simulink model "model_hydrau"  (R2022b)
settings: Solver=VariableStepAuto  StartTime=0.0  StopTime=tmax  MaxStep=2  RelTol=1e-3
values from neighbouring files (symbols this model uses):
  dFmw = 0    [obliczenia.m]    (also in obliczenia2.m)
  k1 = (0.329)/0.0050    (= 65.8)    [obliczenia.m]    (also in obliczenia2.m)
  khC = (91.8012 -90)/0.02    (= 90.06)    [obliczenia.m]
  Kp = 0.9*TczasC/(kC*TopuC)    (= 0.165208580467)    [obliczenia.m]    (also in obliczenia2.m = 1.05226274907)
  Tczas1 = 15543 - Topu1 - tsok    (= 12463)    [obliczenia.m]    (also in obliczenia2.m)
  TczashC = 12982 - Topuh - tsok    (= 9758)    [obliczenia.m]
  Ti = 3.33*TopuC/Kp    (= 13061.3070696)    [obliczenia.m]    (also in obliczenia2.m = 11755.1763626)
  Topu1 = 3080 - tsok    (= 1080)    [obliczenia.m]    (also in obliczenia2.m)
  Topuh = 3224 - tsok    (= 1224)    [obliczenia.m]
  TopuhC = 2740 - tsok    (= 740)    [obliczenia.m]
  TozN = TgzN    (= 90)    [obliczenia.m]    (also in obliczenia2.m)
  tsok = 2000    [obliczenia.m]    (also in obliczenia2.m = 80000)
  Twew10 = (Cpw*Fmg10 *Kcg*Tgz10 + Kcw*(Kcg + Cpw*Fmg10)*Tzew0)/(Kcg*Kcw + Cpw*Fmg10*(Kcg + Kcw))    (= 20)    [obliczenia.m]    (also in obliczenia2.m)
undefined symbols (not defined in the file or in its folder): dTwew
libraries: slpidlib x1
settings Model: Creator=asialalala  LastModifiedBy=asialalala
settings DataIOCC: SaveFormat=Array  ReturnWorkspaceOutputs=off

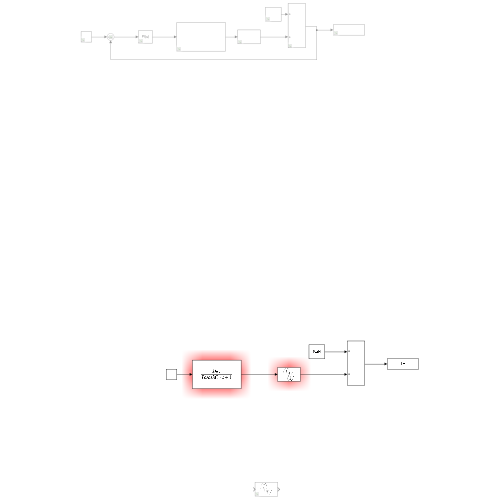
[thumbnail: Simulink's stored preview of the top-level diagram]
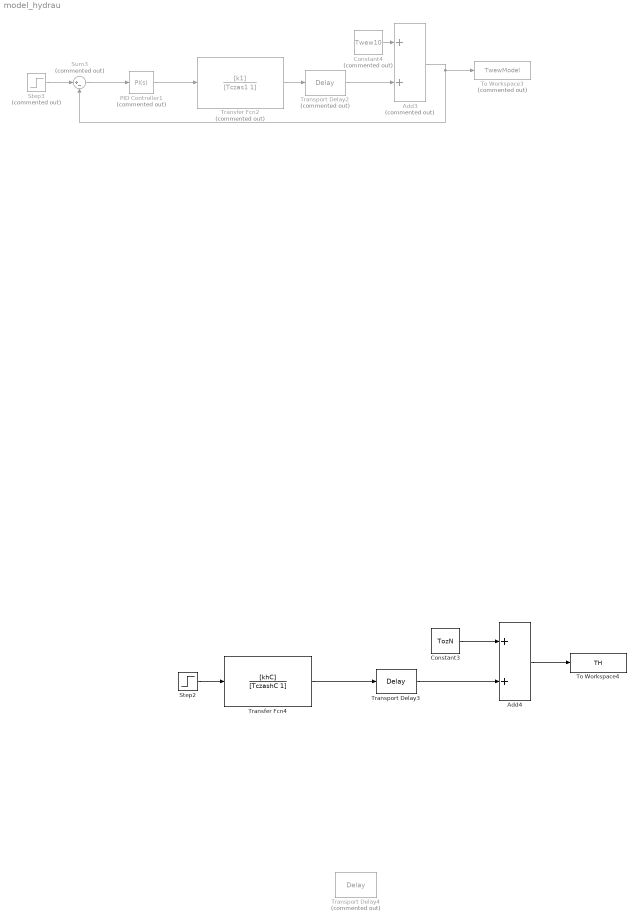
== system model_hydrau ==
  Add3 : Sum  Commented=on
  Add4 : Sum
  Constant3 : Constant  Value=TozN
  Constant4 : Constant  Commented=on  Value=Twew10
  PID Controller1 : slpidlib/PID Controller  Commented=on  Controller=PI  Form=Parallel  TimeDomain=Continuous-time  UseExternalTs=off  SampleTime=-1  IntegratorMethod=Forward Euler  FilterMethod=Forward Euler  ControllerParametersSource=internal  P=Kp  I=1/Ti  UseKiTs=off  D=0  N=100  UseFilter=on  TunerSelectOption=Transfer Function Based (PID Tuner App)  InitialConditionSource=internal  InitialConditionForIntegrator=0  InitialConditionForFilter=0  DifferentiatorICPrevScaledInput=0  ExternalReset=none  TrackingMode=off  Kt=1  LimitOutput=off  SatLimitsSource=internal  UpperSaturationLimit=inf  LowerSaturationLimit=-inf  LinearizeAsGain=on  AntiWindupMode=none  Kb=1  LimitIntegrator=off  UpperIntegratorSaturationLimit=inf  LowerIntegratorSaturationLimit=-inf  POutMin=[]  POutMax=[]  IOutMin=[]  IOutMax=[]  DOutMin=[]  DOutMax=[]  NOutMin=[]  NOutMax=[]  SumOutMin=[]  SumOutMax=[]  SaturationOutMin=[]  SaturationOutMax=[]  PParamMin=[]  PParamMax=[]  IParamMin=[]  IParamMax=[]  DParamMin=[]  DParamMax=[]  NParamMin=[]  NParamMax=[]  KbParamMin=[]  KbParamMax=[]  KtParamMin=[]  KtParamMax=[]  KbOutMin=[]  KbOutMax=[]  KtOutMin=[]  KtOutMax=[]  IntegratorOutMin=[]  IntegratorOutMax=[]  FilterOutMin=[]  FilterOutMax=[]  SumI1OutMin=[]  SumI1OutMax=[]  SumI2OutMin=[]  SumI2OutMax=[]  SumI3OutMin=[]  SumI3OutMax=[]  SumI4OutMin=[]  SumI4OutMax=[]  SumDOutMin=[]  SumDOutMax=[]  DifferentiatorOutMin=[]  DifferentiatorOutMax=[]  FilterDiffOutCoefMin=[]  FilterDiffOutCoefMax=[]  ReciprocalOutMin=[]  ReciprocalOutMax=[]  SumDenOutMin=[]  SumDenOutMax=[]  SumNumOutMin=[]  SumNumOutMax=[]  DivideOutMin=[]  DivideOutMax=[]  UdiffTsProdOutMin=[]  UdiffTsProdOutMax=[]  NTsProdOutMin=[]  NTsProdOutMax=[]  UintegralTsProdOutMin=[]  UintegralTsProdOutMax=[]  UngainTsProdOutMin=[]  UngainTsProdOutMax=[]  ClampingZeroOutDataTypeStr=Inherit: Inherit via back propagation  ClampingZeroOutMin=[]  ClampingZeroOutMax=[]  FilterDenConstantOutDataTypeStr=Inherit: Inherit via back propagation  FilterDenConstantOutMin=[]  FilterDenConstantOutMax=[]  PCopyOutDataTypeStr=Inherit: Inherit via back propagation  PCopyOutMin=[]  PCopyOutMax=[]  NCopyOutDataTypeStr=Inherit: Inherit via back propagation  NCopyOutMin=[]  NCopyOutMax=[]  IntegratorContinuousStateAttributes=''  IntegratorStateMustResolveToSignalObject=off  IntegratorRTWStateStorageClass=Auto  FilterContinuousStateAttributes=''  FilterStateMustResolveToSignalObject=off  FilterRTWStateStorageClass=Auto  ParallelPVariant=InternalParameters  IdealPVariant=Disabled  IVariant=InternalParameters  DVariant=Disabled  IntegratorVariant=Continuous  SatVariant=Disabled  AWVariant=Passthrough  PCopyVariant=Disabled  TRVariant=Disabled  FdbkBlocksVariant=Forward  IdealPFdbkVariant=Disabled  SatFdbkVariant=Disabled  DerivativeFilterVariant=Disabled  NVariant=Disabled  NCopyVariant=Disabled_SignalSpec  FilterICVariant=Disabled  IntegratorICVariant=InternalICs  ExternalResetVariant=Disabled  TRSumVariant=Passthrough  SumFdbkVariant=Disabled  SumVariant=Sum_PI  TsampFilterVariant=InternalTs  TsampNgainVariant=Passthrough  TsampIntegralVariant=Passthrough  ExternalSaturationOutDataTypeStr=Inherit: Same as second input
  Step2 : Step  Time=tsok  After=dFmw  SampleTime=0
  Step3 : Step  Commented=on  Time=tsok  Before=Twew10  After=dTwew + Twew10  SampleTime=0
  Sum3 : Sum  Commented=on  Inputs=|+-
  To Workspace3 : ToWorkspace  Commented=on  VariableName=TwewModel  SampleTime=-1
  To Workspace4 : ToWorkspace  VariableName=TH  SampleTime=-1
  Transfer Fcn2 : TransferFcn  Commented=on  Numerator=[k1]  Denominator=[Tczas1 1]
  Transfer Fcn4 : TransferFcn  Numerator=[khC]  Denominator=[TczashC 1]
  Transport Delay2 : TransportDelay  Commented=on  DelayTime=Topu1
  Transport Delay3 : TransportDelay  DelayTime=TopuhC
  Transport Delay4 : TransportDelay  Commented=on  DelayTime=Topuh
  wires:
  Sum3/1 -> PID Controller1/1
  Transfer Fcn2/1 -> Transport Delay2/1
  Constant4/1 -> Add3/1
  Step3/1 -> Sum3/1
  Add3/1 -> Sum3/2, To Workspace3/1
  PID Controller1/1 -> Transfer Fcn2/1
  Transport Delay2/1 -> Add3/2
  Constant3/1 -> Add4/1
  Add4/1 -> To Workspace4/1
  Step2/1 -> Transfer Fcn4/1
  Transfer Fcn4/1 -> Transport Delay3/1
  Transport Delay3/1 -> Add4/2
